simulink model "swiplInterface"  (R2020b)
settings: Solver=FixedStepAuto  StartTime=0.0  StopTime=10.0  RelTol=1e-3
undefined symbols (not defined in the file or in its folder): AEB
settings Model: Creator=chiar  LastModifiedBy=chiar
settings DebuggingCC: UnknownTsInhSupMsg=none

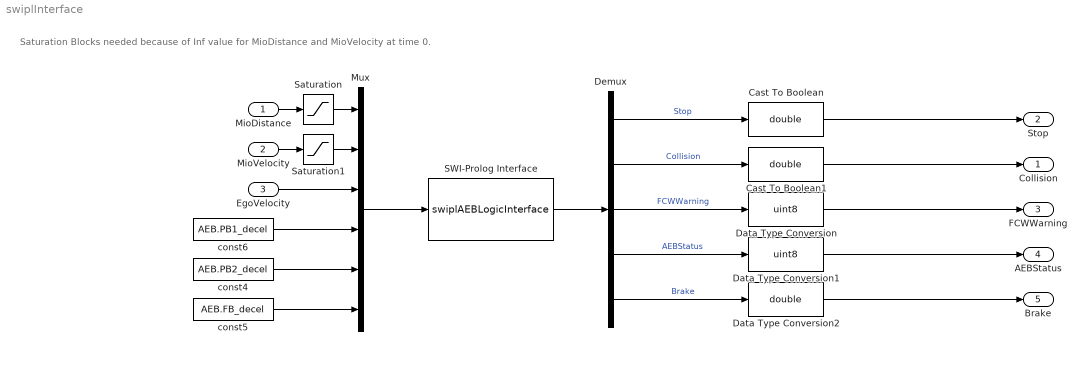
== system swiplInterface ==
  note: Saturation Blocks needed because of Inf value for MioDistance and MioVelocity at time 0.
  MioDistance : Inport
  MioVelocity : Inport  Port=2
  EgoVelocity : Inport  Port=3
  Cast To Boolean : DataTypeConversion  OutDataTypeStr=double
  Cast To Boolean1 : DataTypeConversion  OutDataTypeStr=double
  Data Type Conversion : DataTypeConversion  OutDataTypeStr=uint8
  Data Type Conversion1 : DataTypeConversion  OutDataTypeStr=uint8
  Data Type Conversion2 : DataTypeConversion  OutDataTypeStr=double
  Demux : Demux  Outputs=5
  Mux : Mux  Inputs=6
  SWI-Prolog Interface : S-Function  FunctionName=swiplAEBLogicInterface  Parameters=jplPath, plFile, nIn, plQuery, nOut,0  SFunctionDeploymentMode=off  EnableBusSupport=off  mask(SWI-Prolog (www.swi-prolog.org) Interface){jplPath=C:\Program Files\swipl\lib\jpl.jar, plFile=swiplAEBLogic.pl, nIn=6, nOut=5, plQuery=run(u(1),u(2),u(3),u(4),u(5),u(6),y(1),y(2),y(3),y(4),y(5))}
      mask prompts: jplPath "Path of the JPL jar-file:"; plFile "Prolog file:"; nIn "Number of the inputs:"; nOut "Number of the outputs:"; plQuery "Prolog query:"
      mask help:
      | SWI-Prolog (www.swi-prolog.org) Interface block.
      |
      | Execute Prolog code (PL file) in the Simulink environment.
      |
      | Use ''u'' as the input variable name and ''y'' as the output variable name.
      |
      | In the case of queries with multiple solutions, this block will only return the first solution found.
      mask Help:
      | SWI-Prolog (www.swi-prolog.org) Interface block.
      | 
      | Execute Prolog code (PL file) in the Simulink environment.
      | 
      | Use ''u'' as the input variable name and ''y'' as the output variable name.
      | 
      | In the case of queries with multiple solutions, this block will only return the first solution found.
      mask Display: disp('swipl\nInterface')
  Saturation : Saturate  UpperLimit=10000  LowerLimit=-10000
  Saturation1 : Saturate  UpperLimit=10000  LowerLimit=-10000
  const4 : Constant  Value=AEB.PB2_decel  SampleTime=-1
  const5 : Constant  Value=AEB.FB_decel  SampleTime=-1
  const6 : Constant  Value=AEB.PB1_decel  SampleTime=-1
  Collision : Outport
  Stop : Outport  Port=2
  FCWWarning : Outport  Port=3
  AEBStatus : Outport  Port=4
  Brake : Outport  Port=5
  wires:
  Demux/2 -> Cast To Boolean1/1  "Collision"
  SWI-Prolog Interface/1 -> Demux/1
  MioDistance/1 -> Saturation/1
  Demux/4 -> Data Type Conversion1/1  "AEBStatus"
  Demux/1 -> Cast To Boolean/1  "Stop"
  MioVelocity/1 -> Saturation1/1
  Demux/5 -> Data Type Conversion2/1  "Brake"
  Demux/3 -> Data Type Conversion/1  "FCWWarning"
  EgoVelocity/1 -> Mux/3
  Mux/1 -> SWI-Prolog Interface/1
  const6/1 -> Mux/4
  const4/1 -> Mux/5
  const5/1 -> Mux/6
  Cast To Boolean/1 -> Stop/1
  Cast To Boolean1/1 -> Collision/1
  Data Type Conversion/1 -> FCWWarning/1
  Data Type Conversion1/1 -> AEBStatus/1
  Data Type Conversion2/1 -> Brake/1
  Saturation/1 -> Mux/1
  Saturation1/1 -> Mux/2
